simulink model "CAN_Network"  (R2018a)
settings: Solver=VariableStepAuto  StartTime=0.0  StopTime=10.0  RelTol=1e-3
undefined symbols (not defined in the file): canChannel
libraries: canlib x7, canmsglib x3
settings Model: Creator=SUCHITRA  LastModifiedBy=SUCHITRA

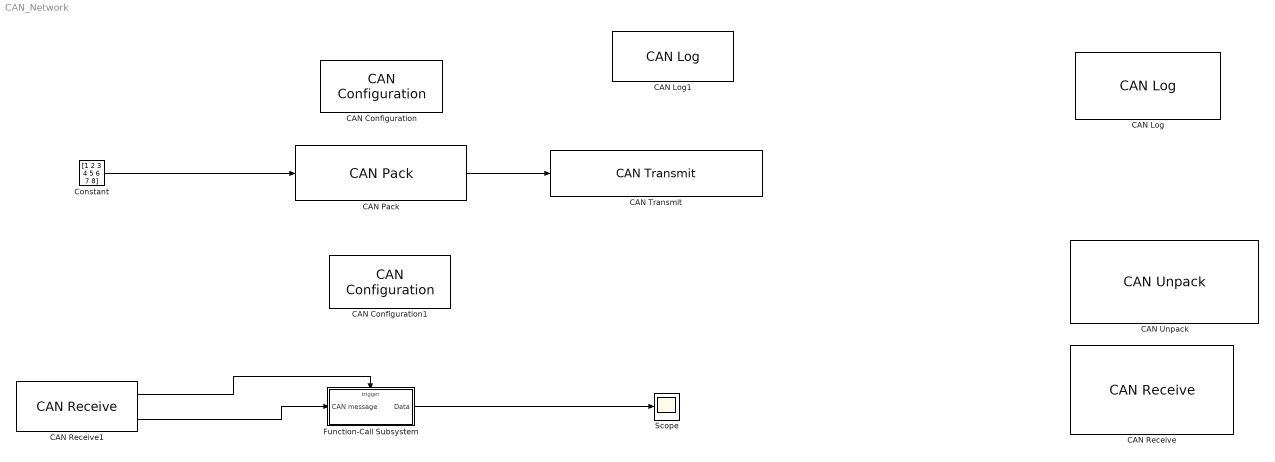
== system CAN_Network ==
  CAN Configuration : canlib/CAN Configuration  BlockHandle=14.0001  DeviceMenu=MathWorks Virtual 1 (Channel 1)  Device=MathWorks Virtual 1 (Channel 1)  ObjConstructor=canChannel('MathWorks','Virtual 1',1)  BusSpeed=250000  EnableBitParameters=off  AckMode=Normal
      settings: SourceProductName=Vehicle Network Toolbox  SourceProductBaseCode=VN
  CAN Configuration1 : canlib/CAN Configuration  BlockHandle=1864.0001  DeviceMenu=MathWorks Virtual 1 (Channel 2)  Device=MathWorks Virtual 1 (Channel 2)  ObjConstructor=canChannel('MathWorks','Virtual 1',2)  BusSpeed=250000  EnableBitParameters=off  AckMode=Normal
      settings: SourceProductName=Vehicle Network Toolbox  SourceProductBaseCode=VN
  CAN Log : canlib/CAN Log  BlockHandle=15.0001  FullPathFileName=untitled.mat  FileName=untitled.mat  VariableName=ans  MaxNumMessages=10000  LogFrom=CAN Bus  DeviceMenu=MathWorks Virtual 1 (Channel 1)  Device=MathWorks Virtual 1 (Channel 1)  ObjConstructor=canChannel('MathWorks','Virtual 1',1)  SampleTime=0.01
      settings: SourceProductName=Vehicle Network Toolbox  SourceProductBaseCode=VN
  CAN Log1 : canlib/CAN Log  BlockHandle=1902.0001  FullPathFileName=CAN_network.mat  FileName=CAN_network.mat  VariableName=ans  MaxNumMessages=10000  LogFrom=CAN Bus  DeviceMenu=MathWorks Virtual 1 (Channel 1)  Device=MathWorks Virtual 1 (Channel 1)  ObjConstructor=canChannel('MathWorks','Virtual 1',1)  SampleTime=0.01
      settings: SourceProductName=Vehicle Network Toolbox  SourceProductBaseCode=VN
  CAN Pack : canmsglib/CAN Pack  MsgList=(none)  MsgName=CAN Msg  MsgIDType=Standard (11-bit identifier)  MsgIdentifier=500  MsgLength=8  NSignals=0  StartBits=0  SignalSizes=0  ByteOrders=0  DataTypes=0  MultiplexTypes=0  MultiplexValues=0  Factors=0  Offsets=0  Minimums=0  Maximums=0  Remote=off  ApplyMinMax=off  BusOutput=off
      settings: SourceProductName=Simulink Real-Time  SourceProductBaseCode=XP  DataFormat=raw data
  CAN Receive : canlib/CAN Receive  BlockHandle=30.0001  DeviceMenu=MathWorks Virtual 1 (Channel 1)  Device=MathWorks Virtual 1 (Channel 1)  ObjConstructor=canChannel('MathWorks','Virtual 1',1)  EnableStandardIDsFilter=off  StandardIDs=0  EnableExtendedIDsFilter=off  ExtendedIDs=0  SampleTime=0.01  MsgsPerTimestep=all  StdIDsCombo=Allow all  ExtIDsCombo=Allow all  InternalFilterUpdateStatus=off  BusOutput=off
      settings: SourceProductName=Vehicle Network Toolbox  SourceProductBaseCode=VN
  CAN Receive1 : canlib/CAN Receive  BlockHandle=1865.0001  DeviceMenu=MathWorks Virtual 1 (Channel 1)  Device=MathWorks Virtual 1 (Channel 1)  ObjConstructor=canChannel('MathWorks','Virtual 1',1)  EnableStandardIDsFilter=off  StandardIDs=0  EnableExtendedIDsFilter=off  ExtendedIDs=0  SampleTime=0.01  MsgsPerTimestep=all  StdIDsCombo=Allow all  ExtIDsCombo=Allow all  InternalFilterUpdateStatus=off  BusOutput=off
      settings: SourceProductName=Vehicle Network Toolbox  SourceProductBaseCode=VN
  CAN Transmit : canlib/CAN Transmit  BlockHandle=1857.0001  DeviceMenu=MathWorks Virtual 1 (Channel 1)  Device=MathWorks Virtual 1 (Channel 1)  ObjConstructor=canChannel('MathWorks','Virtual 1',1)  EnablePeriodicTransmit=off  MessagePeriod=1.000
      settings: SourceProductName=Vehicle Network Toolbox  SourceProductBaseCode=VN
  CAN Unpack : canmsglib/CAN Unpack  MsgName=CAN Msg  MsgIDType=Standard (11-bit identifier)  MsgIdentifier=0  MsgLength=8  NSignals=0  IDPort=off  TimestampPort=off  ErrorPort=off  RemotePort=off  LengthPort=off  StatusPort=off  StartBits=0  SignalSizes=0  ByteOrders=0  DataTypes=0  MultiplexTypes=0  MultiplexValues=0  Factors=0  Offsets=0  Minimums=0  Maximums=0  ApplyMinMax=off
      settings: SourceProductName=Simulink Real-Time  SourceProductBaseCode=XP  DataFormat=raw data
  Constant : Constant  Value=[1 2 3 4 5 6 7 8]  SampleTime=0.01
  Function-Call Subsystem : Subsystem  TreatAsAtomicUnit=on
  Scope : Scope
  wires:
  Constant/1 -> CAN Pack/1
  CAN Pack/1 -> CAN Transmit/1
  CAN Receive1/1 -> Function-Call Subsystem/Trigger
  CAN Receive1/2 -> Function-Call Subsystem/1(CAN message)
  Function-Call Subsystem/1(Data) -> Scope/1

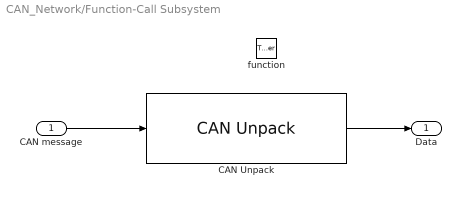
== system CAN_Network/Function-Call Subsystem ==
  CAN message : Inport
  function : TriggerPort  TriggerType=function-call  VariantControl=Variant
  CAN Unpack : canmsglib/CAN Unpack  MsgName=CAN Msg  MsgIDType=Standard (11-bit identifier)  MsgIdentifier=0  MsgLength=8  NSignals=0  IDPort=off  TimestampPort=off  ErrorPort=off  RemotePort=off  LengthPort=off  StatusPort=off  StartBits=0  SignalSizes=0  ByteOrders=0  DataTypes=0  MultiplexTypes=0  MultiplexValues=0  Factors=0  Offsets=0  Minimums=0  Maximums=0  ApplyMinMax=off
      settings: SourceProductName=Simulink Real-Time  SourceProductBaseCode=XP  DataFormat=raw data
  Data : Outport
  wires:
  CAN message/1 -> CAN Unpack/1
  CAN Unpack/1 -> Data/1
